simulink model "mpc_controller"  (R2022b)
settings: Solver=VariableStepAuto  StartTime=0.0  StopTime=10.0  RelTol=1e-3
undefined symbols (not defined in the file or in its folder): m
libraries: mpclib x1
settings Model: Creator=12854  LastModifiedBy=12854

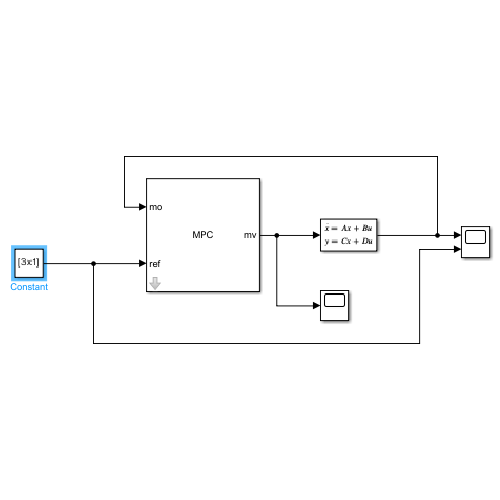
[thumbnail: Simulink's stored preview of the top-level diagram]
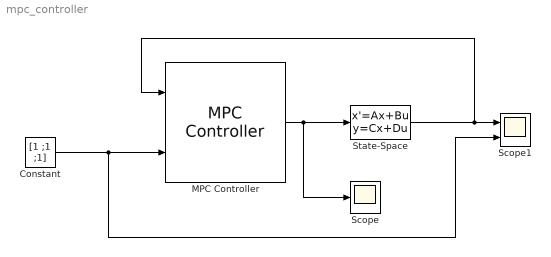
== system mpc_controller ==
  Constant : Constant  Value=[1 ;1 ;1]
  MPC Controller : mpclib/MPC Controller  SCDEnableBlockLinearizationSpecification=on  mpcobj=mpcobj  x0=[]  is_multiple=0  enable_value=0  return_u0=off  updateMPCinCallerWorkspace=on  md_inport=off  mv_inport=off  uref_inport=off  return_cost=off  return_mvseq=off  return_qpstatus=off  return_xseq=off  return_state=off  return_ovseq=off  state_inport=off  umin_inport=off  umax_inport=off  ymin_inport=off  ymax_inport=off  cc_inport=off  ywt_inport=off  uwt_inport=off  duwt_inport=off  rhoeps_inport=off  pm_inport=off  MaximumP=10  HorizonChoice=FixedHorizon  n_ts=0.1  n_p=2  n_mv=3  n_md=0  n_ud=0  n_mo=3  n_uo=0  BlockDataType=double  SampleTimeInherited=off  switch_inport=off
  Scope : Scope
  Scope1 : Scope  NumInputPorts=2
  State-Space : StateSpace  A=[0 0 0 1 0 0; 0 0 0 0 1 0; 0 0 0 0 0 1; 0 0 0 0 0 0; 0 0 0 0 0 0; 0 0 0 0 0 0]  B=[0 0 0; 0 0 0; 0 0 0; 1/m 0 0; 0 1/m 0; 0 0 1/m]  C=[1 0 0 0 0 0; 0 1 0 0 0 0; 0 0 1 0 0 0]  D=zeros(3,3)  InitialCondition=[0; 0; 0; 0; 0; 0]
  wires:
  MPC Controller/1 -> Scope/1, State-Space/1
  State-Space/1 -> MPC Controller/1, Scope1/1
  Constant/1 -> Scope1/2, MPC Controller/2
